simulink model "gifcw_ut"  (Simulink 8.1)
settings: Solver=FixedStepDiscrete  StartTime=0.0  StopTime=10.0  FixedStep=5E-3  RelTol=1e-3
libraries: siltestlib x10, idiada_lib x4, gifcw x1
settings Model: Creator=xsellart  LastModifiedBy=AT015555
settings DataIOCC: SignalLoggingSaveFormat=Dataset
settings OptimizationCC: ExpressionDepthLimit=128
settings DebuggingCC: FcnCallInpInsideContextMsg=EnableAllAsError
settings GRTTargetCC: CombineOutputUpdateFcns=on  GRTInterface=off

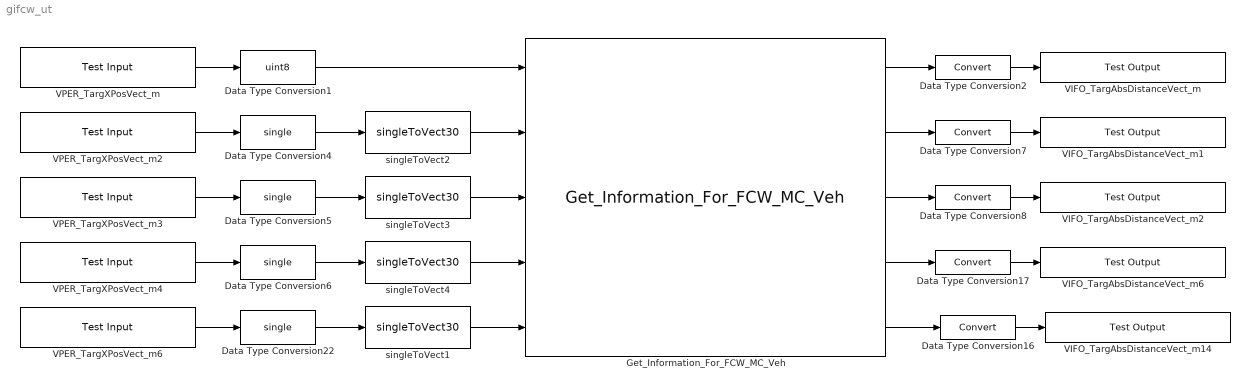
== system gifcw_ut ==
  Data Type Conversion1 : DataTypeConversion  OutDataTypeStr=uint8
  Data Type Conversion{2,7..8,16..17} (5 alike) : DataTypeConversion
  Data Type Conversion{4..6,22} (4 alike) : DataTypeConversion  OutDataTypeStr=single
  Get_Information_For_FCW_MC_Veh : gifcw/Get_Information_For_FCW_MC_Veh
  VIFO_TargAbsDistanceVect_m : siltestlib/Test Output  varname=NIFO_FCWTargetVehRelSpeedX_mps  sampletime=-1
  VIFO_TargAbsDistanceVect_m1 : siltestlib/Test Output  varname=NIFO_FCWMCVehXPosition_m  sampletime=-1
  VIFO_TargAbsDistanceVect_m14 : siltestlib/Test Output  varname=NIFO_FCWMCLongAccel_mps2  sampletime=-1
  VIFO_TargAbsDistanceVect_m2 : siltestlib/Test Output  varname=NIFO_FCWTargetVehAssigned_flg  sampletime=-1
  VIFO_TargAbsDistanceVect_m6 : siltestlib/Test Output  varname=NIFO_FCWMCVehId_num  sampletime=-1
  VPER_TargXPosVect_m : siltestlib/Test Input  varname=VIFO_FCWMCTTargetId_num  sampletime=0.005
  VPER_TargXPosVect_m2 : siltestlib/Test Input  varname=VPER_TargXPosVect30_m  sampletime=0.005
  VPER_TargXPosVect_m3 : siltestlib/Test Input  varname=VIFO_TargVehRelSpdXVect30_mps  sampletime=0.005
  VPER_TargXPosVect_m4 : siltestlib/Test Input  varname=VPER_TargIdVect30_num  sampletime=0.005
  VPER_TargXPosVect_m6 : siltestlib/Test Input  varname=VIFO_TargAccelXVect30_mps2  sampletime=0.005
  singleToVect{1..4} (4 alike) : idiada_lib/singleToVect30
  wires:
  VPER_TargXPosVect_m/1 -> Data Type Conversion1/1
  Data Type Conversion1/1 -> Get_Information_For_FCW_MC_Veh/1
  Get_Information_For_FCW_MC_Veh/1 -> Data Type Conversion2/1
  Data Type Conversion2/1 -> VIFO_TargAbsDistanceVect_m/1
  VPER_TargXPosVect_m2/1 -> Data Type Conversion4/1
  Data Type Conversion4/1 -> singleToVect2/1
  VPER_TargXPosVect_m3/1 -> Data Type Conversion5/1
  Data Type Conversion5/1 -> singleToVect3/1
  VPER_TargXPosVect_m4/1 -> Data Type Conversion6/1
  Data Type Conversion6/1 -> singleToVect4/1
  Get_Information_For_FCW_MC_Veh/2 -> Data Type Conversion7/1
  Data Type Conversion7/1 -> VIFO_TargAbsDistanceVect_m1/1
  Get_Information_For_FCW_MC_Veh/3 -> Data Type Conversion8/1
  Data Type Conversion8/1 -> VIFO_TargAbsDistanceVect_m2/1
  singleToVect2/1 -> Get_Information_For_FCW_MC_Veh/2
  singleToVect3/1 -> Get_Information_For_FCW_MC_Veh/3
  singleToVect4/1 -> Get_Information_For_FCW_MC_Veh/4
  Data Type Conversion17/1 -> VIFO_TargAbsDistanceVect_m6/1
  Data Type Conversion16/1 -> VIFO_TargAbsDistanceVect_m14/1
  Get_Information_For_FCW_MC_Veh/4 -> Data Type Conversion17/1
  Get_Information_For_FCW_MC_Veh/5 -> Data Type Conversion16/1
  VPER_TargXPosVect_m6/1 -> Data Type Conversion22/1
  Data Type Conversion22/1 -> singleToVect1/1
  singleToVect1/1 -> Get_Information_For_FCW_MC_Veh/5
